simulink model "a1_Conventional_EUROPE_1s_C_18b"  (R2018b)
settings: Solver=VariableStepAuto  StartTime=0  StopTime=80  RelTol=1e-3
values from neighbouring files (symbols this model uses):
  E_load = 150    [a1_Conventional_mechlimit_EUR.m]    (also in calc_criticaltime.m; calc_nadir_IBFPR_SI.m; calc_variables_a1Ta.m; power_reserve.m)
  H = Ek/Sb    (= 0.375)    [a1_Conventional_mechlimit_EUR.m]    (also in calc_criticaltime.m = 3.75; calc_nadir_IBFPR_SI.m = 1.035; calc_variables_a1Ta.m = 2.25; power_reserve.m = 3.75)
  Sb = 200    [a1_Conventional_mechlimit_EUR.m]    (also in calc_criticaltime.m; calc_nadir_IBFPR_SI.m = 166.666666667; calc_variables_a1Ta.m = 166.666666667; power_reserve.m)
  T_1 = data1(2)    [a1_Conventional_mechlimit_EUR.m]    (also in calc_criticaltime.m; calc_nadir_IBFPR_SI.m; calc_variables_a1Ta.m; power_reserve.m)
  T_2 = data1(3)    [a1_Conventional_mechlimit_EUR.m]    (also in calc_criticaltime.m; calc_nadir_IBFPR_SI.m; calc_variables_a1Ta.m; power_reserve.m)
  T_3 = data1(4)    [a1_Conventional_mechlimit_EUR.m]    (also in calc_criticaltime.m; calc_nadir_IBFPR_SI.m; calc_variables_a1Ta.m; power_reserve.m)
  T_4 = data1(5)    [a1_Conventional_mechlimit_EUR.m]    (also in calc_criticaltime.m; calc_nadir_IBFPR_SI.m; calc_variables_a1Ta.m; power_reserve.m)
  un = 0.02    [calc_nadir_IBFPR_SI.m]    (also in calc_variables_a1Ta.m)
settings Model: Creator=estuser04  LastModifiedBy=Alejandro
settings SolverCC: AlgebraicLoopSolver=LineSearch

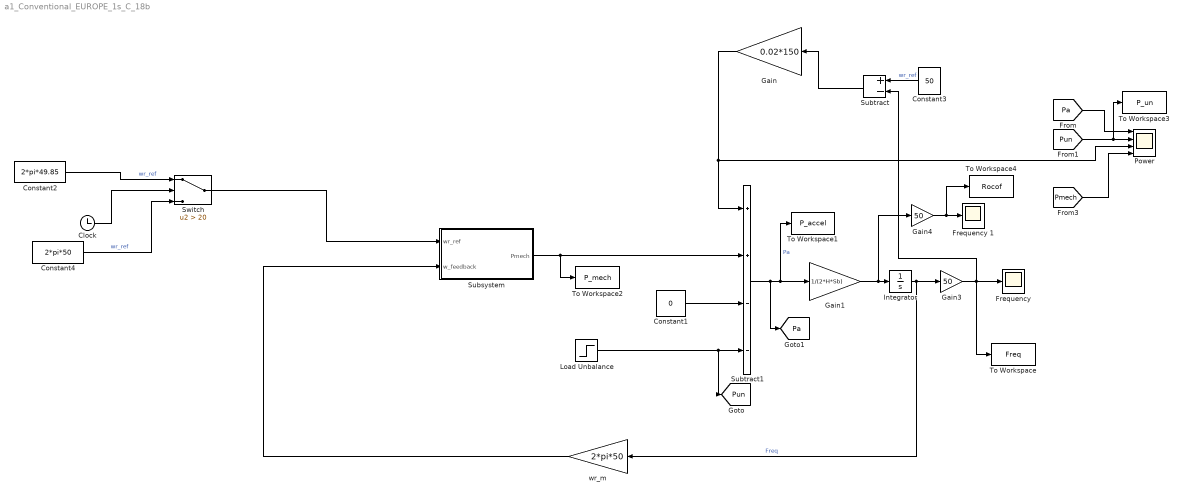
== system a1_Conventional_EUROPE_1s_C_18b ==
  Clock : Clock
  Constant1 : Constant  Value=0
  Constant2 : Constant  Value=2*pi*49.85
  Constant3 : Constant  Value=50
  Constant4 : Constant  Value=2*pi*50
  "Frequency " : Scope
  Frequency 1 : Scope
  Gain : Gain  Gain=0.02*150
  Gain1 : Gain  Gain=1/(2*H*Sb)
  Gain3 : Gain  Gain=50
  Gain4 : Gain  Gain=50
  Integrator : Integrator  InitialCondition=1
  Load Unbalance : Step  Time=0  After=E_load*un  SampleTime=0
  Power : Scope  NumInputPorts=4
  Subsystem : Subsystem
  Subtract : Sum  Inputs=+-
  Subtract1 : Sum  Inputs=++--
  Switch : Switch  Criteria=u2 > Threshold  Threshold=20
  To Workspace : ToWorkspace  VariableName=Freq  SaveFormat=Timeseries  SampleTime=-1
  To Workspace1 : ToWorkspace  VariableName=P_accel  SaveFormat=Timeseries  SampleTime=-1
  To Workspace2 : ToWorkspace  VariableName=P_mech  SaveFormat=Timeseries  SampleTime=-1
  To Workspace3 : ToWorkspace  VariableName=P_un  SaveFormat=Timeseries  SampleTime=-1
  To Workspace4 : ToWorkspace  VariableName=Rocof  SaveFormat=Timeseries  SampleTime=-1
  "wr_m " : Gain  Gain=2*pi*50
  tag scope: Pa=global, Pun=global
  wires:
  Integrator/1 -> Gain3/1, "wr_m "/1  "Freq"
  Subtract1/1 -> [Pa], To Workspace1/1, Gain1/1  "Pa"
  Constant1/1 -> Subtract1/3
  Constant2/1 -> Switch/1  "wr_ref"
  "wr_m "/1 -> Subsystem/2(w_feedback)
  Subsystem/1(Pmech) -> To Workspace2/1, Subtract1/2
  [Pa] -> Power/1
  [Pun] -> To Workspace3/1, Power/2
  [Pmech] -> Power/4
  Gain1/1 -> Gain4/1, Integrator/1
  Gain4/1 -> To Workspace4/1, Frequency 1/1
  Constant3/1 -> Subtract/1  "wr_ref"
  Subtract/1 -> Gain/1
  Gain3/1 -> Subtract/2, To Workspace/1, "Frequency "/1
  Gain/1 -> Subtract1/1, Power/3
  Load Unbalance/1 -> [Pun], Subtract1/4
  Constant4/1 -> Switch/3  "wr_ref"
  Clock/1 -> Switch/2
  Switch/1 -> Subsystem/1(wr_ref)

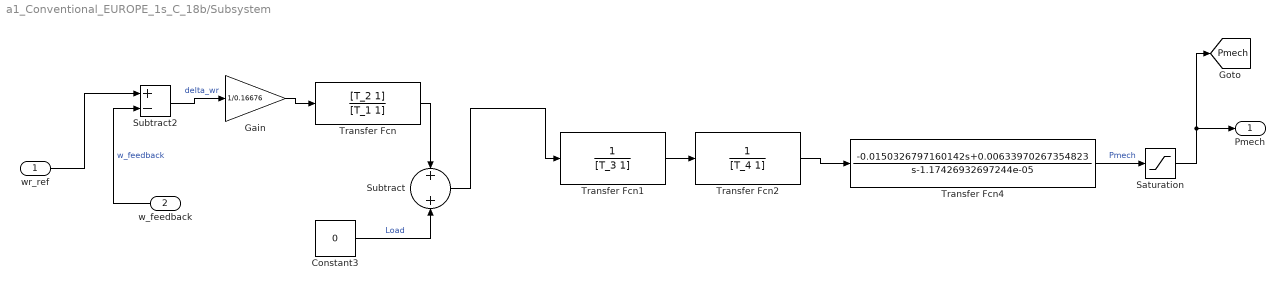
== system a1_Conventional_EUROPE_1s_C_18b/Subsystem ==
  wr_ref : Inport
  w_feedback : Inport  Port=2
  Constant3 : Constant  Value=0
  Gain : Gain  Gain=1/0.16676
  Saturation : Saturate  UpperLimit=un*E_load  LowerLimit=0
  Subtract : Sum
  Subtract2 : Sum  Inputs=+-
  Transfer Fcn : TransferFcn  Numerator=[T_2 1]  Denominator=[T_1 1]
  Transfer Fcn1 : TransferFcn  Denominator=[T_3 1]
  Transfer Fcn2 : TransferFcn  Denominator=[T_4 1]
  Transfer Fcn4 : TransferFcn  Numerator=[-0.0150326797160142 0.00633970267354823]  Denominator=[1 -1.17426932697244e-05]
  Pmech : Outport
  tag scope: Pmech=global
  wires:
  Constant3/1 -> Subtract/2  "Load"
  Transfer Fcn/1 -> Subtract/1
  Gain/1 -> Transfer Fcn/1
  Transfer Fcn2/1 -> Transfer Fcn4/1
  w_feedback/1 -> Subtract2/2  "w_feedback"
  Transfer Fcn1/1 -> Transfer Fcn2/1
  wr_ref/1 -> Subtract2/1
  Transfer Fcn4/1 -> Saturation/1  "Pmech"
  Subtract2/1 -> Gain/1  "delta_wr"
  Subtract/1 -> Transfer Fcn1/1
  Saturation/1 -> [Pmech], Pmech/1
